simulink model "dpt_velosity"  (R2021b)
settings: Solver=VariableStepAuto  StartTime=0.0  StopTime=0.5  RelTol=1e-3
values from neighbouring files (symbols this model uses):
  Jn = 2*Jd    (= 3.92e-05)    [pasport_dpt.m]
  ke = (Un-R*In)/wn    (= 0.236312997347)    [pasport_dpt.m]
  km = Mn/In    (= 0.156097560976)    [pasport_dpt.m]
  ku = 20    [pasport_dpt.m]
  R = 51    [pasport_dpt.m]
  Te = L/R    (= 0.00274509803922)    [pasport_dpt.m]
settings Model: Creator=Admin  LastModifiedBy=Admin
settings SolverCC: AlgebraicLoopSolver=TrustRegion
settings DebuggingCC: SFMachineParentedDataDiag=warning

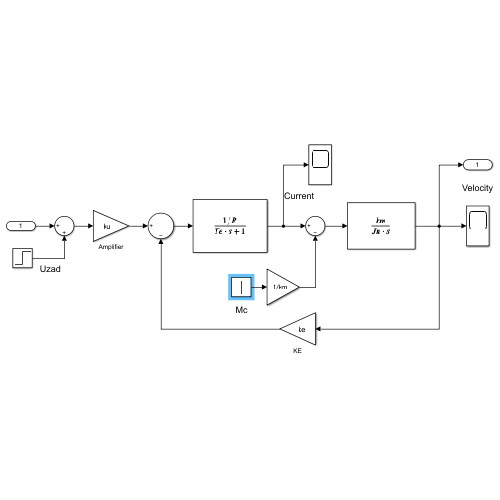
[thumbnail: Simulink's stored preview of the top-level diagram]
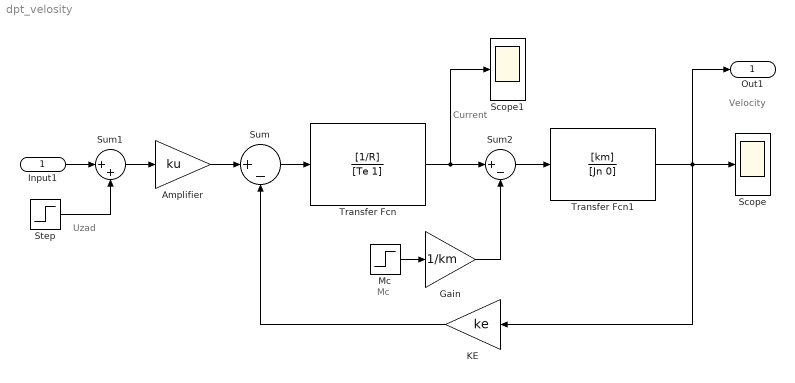
== system dpt_velosity ==
  note: Uzad
  note: Mc
  note: Velocity
  note: Current
  Input1 : Inport
  Amplifier : Gain  Gain=ku
  Gain : Gain  Gain=1/km
  KE : Gain  Gain=ke
  Mc : Step  Time=0.35  After=0.02  SampleTime=0  ZeroCross=off
  Scope : Scope
  Scope1 : Scope
  Step : Step  Time=0  SampleTime=0  ZeroCross=off
  Sum : Sum  Inputs=|+-
  Sum1 : Sum  Inputs=|++
  Sum2 : Sum  Inputs=|+-
  Transfer Fcn : TransferFcn  Numerator=[1/R]  Denominator=[Te 1]
  Transfer Fcn1 : TransferFcn  Numerator=[km]  Denominator=[Jn 0]
  Out1 : Outport  BusOutputAsStruct=on
  wires:
  Amplifier/1 -> Sum/1
  Input1/1 -> Sum1/1
  Sum1/1 -> Amplifier/1
  KE/1 -> Sum/2
  Step/1 -> Sum1/2
  Sum/1 -> Transfer Fcn/1
  Transfer Fcn/1 -> Sum2/1, Scope1/1
  Sum2/1 -> Transfer Fcn1/1
  Transfer Fcn1/1 -> KE/1, Out1/1, Scope/1
  Gain/1 -> Sum2/2
  Mc/1 -> Gain/1
